simulink model "LQR"  (R2021a)
settings: Solver=VariableStepAuto  StartTime=0.0  StopTime=10.0  RelTol=1e-3
settings Model: Creator=SHUDaXIA  LastModifiedBy=SHUDaXIA

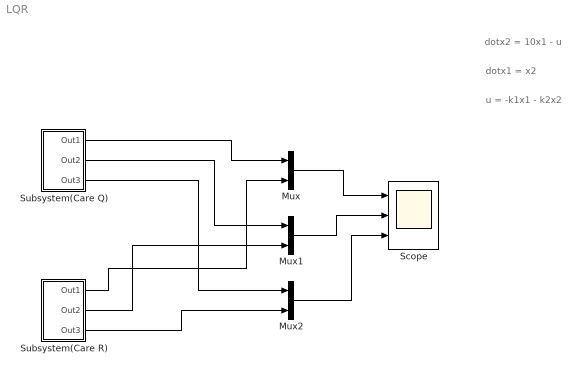
== system LQR ==
  note: u = -k1x1 - k2x2
  note: dotx1 = x2
  note: dotx2 = 10x1 - u
  Mux : Mux  Inputs=2
  Mux1 : Mux  Inputs=2
  Mux2 : Mux  Inputs=2
  Scope : Scope  NumInputPorts=3
  Subsystem(Care Q) : Subsystem
  Subsystem(Care R) : Subsystem
  wires:
  Subsystem(Care Q)/1(Out1) -> Mux/1
  Subsystem(Care Q)/2(Out2) -> Mux1/1
  Subsystem(Care Q)/3(Out3) -> Mux2/1
  Subsystem(Care R)/1(Out1) -> Mux/2
  Subsystem(Care R)/2(Out2) -> Mux1/2
  Subsystem(Care R)/3(Out3) -> Mux2/2
  Mux/1 -> Scope/1
  Mux1/1 -> Scope/2
  Mux2/1 -> Scope/3

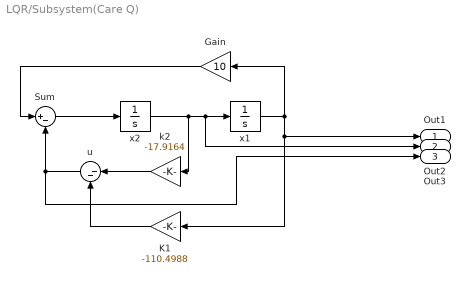
== system LQR/Subsystem(Care Q) ==
  Gain : Gain  Gain=10
  K1 : Gain  Gain=-110.4988
  Sum : Sum  Inputs=|+-
  k2 : Gain  Gain=-17.9164
  u : Sum  Inputs=|--
  x1 : Integrator  InitialCondition=5
  x2 : Integrator
  Out1 : Outport
  Out2 : Outport  Port=2
  Out3 : Outport  Port=3
  wires:
  k2/1 -> u/1
  x2/1 -> k2/1, Out2/1, x1/1
  x1/1 -> Out1/1, K1/1, Gain/1
  u/1 -> Out3/1, Sum/2
  K1/1 -> u/2
  Sum/1 -> x2/1
  Gain/1 -> Sum/1

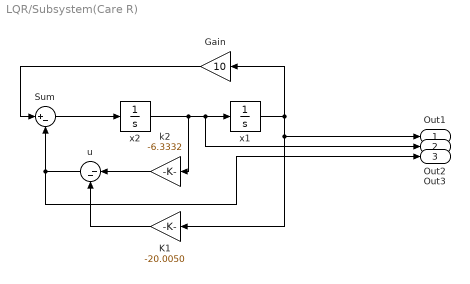
== system LQR/Subsystem(Care R) ==
  Gain : Gain  Gain=10
  K1 : Gain  Gain=-20.0050
  Sum : Sum  Inputs=|+-
  k2 : Gain  Gain=-6.3332
  u : Sum  Inputs=|--
  x1 : Integrator  InitialCondition=5
  x2 : Integrator
  Out1 : Outport
  Out2 : Outport  Port=2
  Out3 : Outport  Port=3
  wires:
  Gain/1 -> Sum/1
  Sum/1 -> x2/1
  K1/1 -> u/2
  u/1 -> Sum/2, Out3/1
  x1/1 -> Gain/1, K1/1, Out1/1
  x2/1 -> x1/1, Out2/1, k2/1
  k2/1 -> u/1
